simulink model "zad71_tran"  (R2015a)
settings: Solver=FixedStepDiscrete  StartTime=0.0  StopTime=99.0  FixedStep=1  RelTol=1e-3
settings Model: Creator=Bojana Vasic  LastModifiedBy=Bojana Vasic

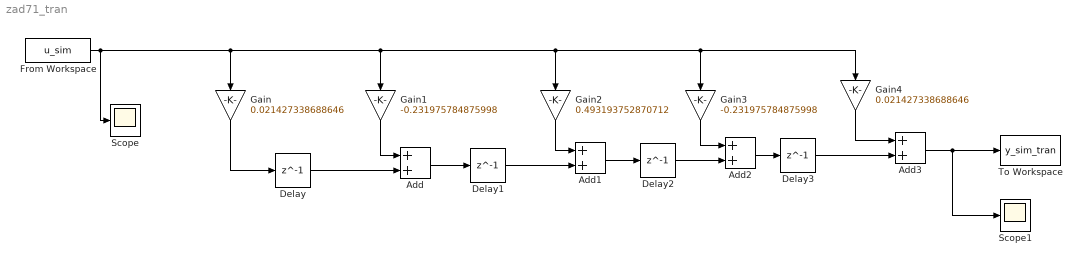
== system zad71_tran ==
  Add{,1..3} (4 alike) : Sum
  Delay{,1..3} (4 alike) : Delay  DelayLength=1
  From Workspace : FromWorkspace  VariableName=u_sim  SampleTime=1
  Gain : Gain  Gain=0.021427338688646
  Gain1 : Gain  Gain=-0.231975784875998
  Gain2 : Gain  Gain=0.493193752870712
  Gain3 : Gain  Gain=-0.231975784875998
  Gain4 : Gain  Gain=0.021427338688646
  Scope : Scope
  Scope1 : Scope
  To Workspace : ToWorkspace  VariableName=y_sim_tran  SampleTime=-1
      settings: Save2DSignal=2-D array (concatenate along first dimension)
  wires:
  From Workspace/1 -> Scope/1, Gain4/1, Gain3/1, Gain2/1, Gain1/1, Gain/1
  Gain1/1 -> Add/1
  Gain2/1 -> Add1/1
  Gain3/1 -> Add2/1
  Gain4/1 -> Add3/1
  Add3/1 -> Scope1/1, To Workspace/1
  Add2/1 -> Delay3/1
  Gain/1 -> Delay/1
  Delay/1 -> Add/2
  Add/1 -> Delay1/1
  Delay1/1 -> Add1/2
  Add1/1 -> Delay2/1
  Delay2/1 -> Add2/2
  Delay3/1 -> Add3/2
